simulink subsystem "shading_array"  (R2025a)
settings: Solver=VariableStepAuto  StartTime=0.0  StopTime=10.0  RelTol=1e-3
libraries: spsDiodeLib x5, spsPVArrayLib x5, spsSeriesRLCBranchLib x5, eeGeneralControl x3, spsCurrentMeasurementLib x1, spsGroundLib x1, spsVoltageMeasurementLib x1
settings Model: Creator=harsh  LastModifiedBy=harsh

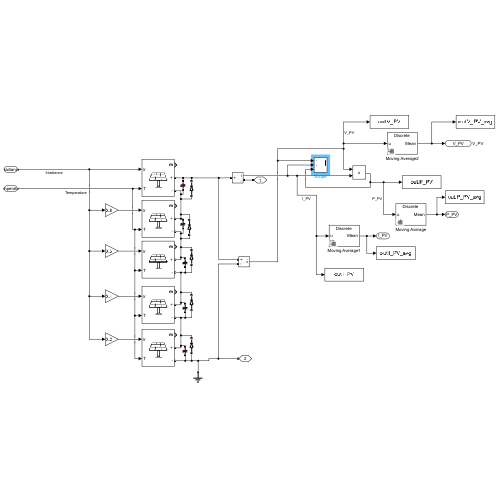
[thumbnail: Simulink's stored preview of the top-level diagram]
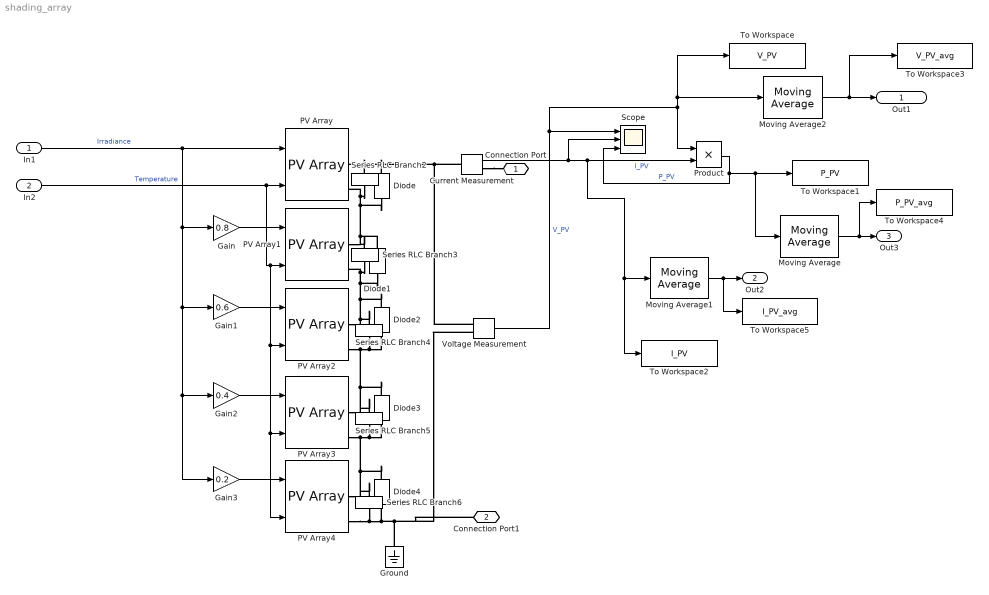
== system shading_array ==
  In1 : Inport
  In2 : Inport  Port=2
  Current Measurement : spsCurrentMeasurementLib/Current Measurement  PhasorSimulation=off  OutputType=Complex  PSBequivalent=0
  Diode{,1..4} (5 alike) : spsDiodeLib/Diode  Ron=0.001  Lon=0  Vf=0.8  IC=0  UseSnubber=0  Rs=inf  Cs=0  Measurements=off
  Gain : Gain  Gain=0.8
  Gain1 : Gain  Gain=0.6
  Gain2 : Gain  Gain=0.4
  Gain3 : Gain  Gain=0.2
  Ground : spsGroundLib/Ground  LConnTagsString=a
  Moving Average : eeGeneralControl/Moving Average  VariantControl=Variant1  LabelModeActiveChoice=Discrete  f=100  x0=0  BufferSize=8192  Ts=-1
      settings: LibrarySourceBlock=ee_sl_lib/General Control/Moving Average
  Moving Average1 : eeGeneralControl/Moving Average  VariantControl=Variant1  LabelModeActiveChoice=Discrete  f=100  x0=0  BufferSize=8192  Ts=-1
      settings: LibrarySourceBlock=ee_sl_lib/General Control/Moving Average
  Moving Average2 : eeGeneralControl/Moving Average  VariantControl=Variant1  LabelModeActiveChoice=Discrete  f=100  x0=0  BufferSize=8192  Ts=-1
      settings: LibrarySourceBlock=ee_sl_lib/General Control/Moving Average
  PV Array{,1..4} (5 alike) : spsPVArrayLib/PV Array  Npar=1  Nser=1  PlotType=one module @ 25 deg.C & specified irradiances  S_vec="[ 1000  500  100 ]"  Temp_C_vec="[ 45 25  ]"  ModuleName=A10Green Technology A10J-S72-175  PlotWhenSelected=off  Pm=175.0914  Ncell=72  Voc=43.99  Isc=5.17  Vm=36.63  Im=4.78  beta_Voc_pc=-0.3616  alpha_Isc_pc=0.041509  beta_Voc=-0.15907  alpha_Isc=0.002146  IL=5.178  I0=1.7842e-10  nI=0.98852  Rsh=249.6758  Rs=0.38412  RobustModel=off  RobustCellTemperature=313.3991  BAL=on  Tc=1e-6  Tfilter=5e-5
  Product : Product
  Scope : Scope  NumInputPorts=3
      settings: ActiveDisplayYMinimum=-26.679627518647923  ActiveDisplayYMaximum=240.14887143716567  DataLoggingVariableName=ScopeData5
  Series RLC Branch{2..6} (5 alike) : spsSeriesRLCBranchLib/Series RLC Branch  LConnTagsString=__new0  RConnTagsString=__new0  BranchType=C  Resistance=23  Inductance=0  SetiL0=off  InitialCurrent=0  Capacitance=1e-6  Setx0=off  InitialVoltage=0  Measurements=None
  To Workspace : ToWorkspace  VariableName=V_PV  SampleTime=-1
  To Workspace1 : ToWorkspace  VariableName=P_PV  SampleTime=-1
  To Workspace2 : ToWorkspace  VariableName=I_PV  SampleTime=-1
  To Workspace3 : ToWorkspace  VariableName=V_PV_avg  SampleTime=-1
  To Workspace4 : ToWorkspace  VariableName=P_PV_avg  SampleTime=-1
  To Workspace5 : ToWorkspace  VariableName=I_PV_avg  SampleTime=-1
  Voltage Measurement : spsVoltageMeasurementLib/Voltage Measurement  PhasorSimulation=off  OutputType=Complex  PSBequivalent=0
  Connection Port : PMIOPort  Side=Right
  Connection Port1 : PMIOPort  Port=2  Side=Left
  Out1 : Outport  SignalName=V_PV
  Out2 : Outport  Port=2
  Out3 : Outport  Port=3
  wires:
  Current Measurement/1 -> Scope/2, To Workspace2/1, Moving Average1/1, Product/2  "I_PV"
  Gain1/1 -> PV Array2/1
  Gain3/1 -> PV Array4/1
  Product/1 -> Scope/3, To Workspace1/1, Moving Average/1  "P_PV"
  In2/1 -> PV Array4/2, PV Array3/2, PV Array2/2, PV Array1/2, PV Array/2  "Temperature"
  Gain/1 -> PV Array1/1
  Voltage Measurement/1 -> To Workspace/1, Moving Average2/1, Product/1, Scope/1  "V_PV"
  In1/1 -> Gain3/1, Gain2/1, Gain1/1, Gain/1, PV Array/1  "Irradiance"
  Gain2/1 -> PV Array3/1
  Moving Average/1 -> To Workspace4/1, Out3/1
  Moving Average1/1 -> To Workspace5/1, Out2/1
  Moving Average2/1 -> To Workspace3/1, Out1/1
  connections:
  Series RLC Branch5/RConn1 -- PV Array4/RConn1 -- Series RLC Branch6/LConn1 -- Diode4/RConn1 -- PV Array3/RConn2 -- Diode3/LConn1
  PV Array4/RConn2 -- Voltage Measurement/LConn2 -- Connection Port1/RConn1 -- Ground/LConn1 -- Diode4/LConn1 -- Series RLC Branch6/RConn1
  Series RLC Branch4/RConn1 -- PV Array3/RConn1 -- Series RLC Branch5/LConn1 -- Diode3/RConn1 -- PV Array2/RConn2 -- Diode2/LConn1
  PV Array2/RConn1 -- Series RLC Branch3/RConn1 -- PV Array1/RConn2 -- Diode1/LConn1 -- Diode2/RConn1 -- Series RLC Branch4/LConn1
  Current Measurement/LConn1 -- Series RLC Branch2/LConn1 -- PV Array/RConn1 -- Diode/RConn1 -- Voltage Measurement/LConn1
  Series RLC Branch2/RConn1 -- PV Array1/RConn1 -- Series RLC Branch3/LConn1 -- Diode1/RConn1 -- Diode/LConn1 -- PV Array/RConn2
  Current Measurement/RConn1 -- Connection Port/RConn1
